simulink model "Model"  (R2020b)
settings: Solver=FixedStepDiscrete  StartTime=0.0  StopTime=inf  RelTol=1e-3
undefined symbols (not defined in the file): C12, designMultirateFIR, dt0
libraries: dspmlti4 x96, dspsrcs4 x89
(part 3 of 6)

== system Model/CORE_3_5/Path5 ==
  <IQ> : Inport
  Complex to Real-Imag : ComplexToRealImag
  Complex to Real-Imag1 : ComplexToRealImag
  Constant : Constant  Value=C12  SampleTime=dt0
  DDS_Gen1 : Subsystem
  FIR Dec1 : dspmlti4/FIR Decimation  FilterSource=Input port  h=designMultirateFIR(1,2)  D=2  filtStruct=Direct form  FilterObject=FDECIM  framing=Allow multirate processing  inputOffset=0  outputBufInitCond=0  roundingMode=Floor  overflowMode=off  firstCoeffDataTypeStr=Inherit: Same word length as input  firstCoeffMin=[]  firstCoeffMax=[]  firstCoeffLastDataTypeStr=Inherit: Same word length as input  outputDataTypeStr=Inherit: Same as accumulator  outputMin=[]  outputMax=[]  outputLastDataTypeStr=Inherit: Same as accumulator
  Freq1 : Constant  Value=2.4e6
  Mixer1 : Subsystem
  Real-Imag to Complex : RealImagToComplex
  Out1 : Outport
  wires:
  Constant/1 -> FIR Dec1/2
  Complex to Real-Imag/1 -> Mixer1/1(Input_I)
  Complex to Real-Imag1/1 -> Mixer1/3(DDS_I)
  Mixer1/2(Output_Q) -> Real-Imag to Complex/2
  Freq1/1 -> DDS_Gen1/1(In1)
  Complex to Real-Imag/2 -> Mixer1/2(Input_Q)
  Complex to Real-Imag1/2 -> Mixer1/4(DDS_Q)
  DDS_Gen1/1(Out1) -> Complex to Real-Imag1/1
  Real-Imag to Complex/1 -> FIR Dec1/1
  Mixer1/1(Output_I) -> Real-Imag to Complex/1
  FIR Dec1/1 -> Out1/1
  <IQ>/1 -> Complex to Real-Imag/1

== system Model/CORE_3_5/Path6 ==
  <IQ> : Inport
  Complex to Real-Imag : ComplexToRealImag
  Complex to Real-Imag1 : ComplexToRealImag
  Constant : Constant  Value=C12  SampleTime=dt0
  DDS_Gen1 : Subsystem
  FIR Dec1 : dspmlti4/FIR Decimation  FilterSource=Input port  h=designMultirateFIR(1,2)  D=2  filtStruct=Direct form  FilterObject=FDECIM  framing=Allow multirate processing  inputOffset=0  outputBufInitCond=0  roundingMode=Floor  overflowMode=off  firstCoeffDataTypeStr=Inherit: Same word length as input  firstCoeffMin=[]  firstCoeffMax=[]  firstCoeffLastDataTypeStr=Inherit: Same word length as input  outputDataTypeStr=Inherit: Same as accumulator  outputMin=[]  outputMax=[]  outputLastDataTypeStr=Inherit: Same as accumulator
  Freq1 : Constant  Value=2.4e6
  Mixer1 : Subsystem
  Real-Imag to Complex : RealImagToComplex
  Out1 : Outport
  wires:
  Constant/1 -> FIR Dec1/2
  Complex to Real-Imag/1 -> Mixer1/1(Input_I)
  Complex to Real-Imag1/1 -> Mixer1/3(DDS_I)
  Mixer1/2(Output_Q) -> Real-Imag to Complex/2
  Freq1/1 -> DDS_Gen1/1(In1)
  Complex to Real-Imag/2 -> Mixer1/2(Input_Q)
  Complex to Real-Imag1/2 -> Mixer1/4(DDS_Q)
  DDS_Gen1/1(Out1) -> Complex to Real-Imag1/1
  Real-Imag to Complex/1 -> FIR Dec1/1
  Mixer1/1(Output_I) -> Real-Imag to Complex/1
  FIR Dec1/1 -> Out1/1
  <IQ>/1 -> Complex to Real-Imag/1

== system Model/CORE_3_5/Path7 ==
  <IQ> : Inport
  Complex to Real-Imag : ComplexToRealImag
  Complex to Real-Imag1 : ComplexToRealImag
  Constant : Constant  Value=C12  SampleTime=dt0
  DDS_Gen1 : Subsystem
  FIR Dec1 : dspmlti4/FIR Decimation  FilterSource=Input port  h=designMultirateFIR(1,2)  D=2  filtStruct=Direct form  FilterObject=FDECIM  framing=Allow multirate processing  inputOffset=0  outputBufInitCond=0  roundingMode=Floor  overflowMode=off  firstCoeffDataTypeStr=Inherit: Same word length as input  firstCoeffMin=[]  firstCoeffMax=[]  firstCoeffLastDataTypeStr=Inherit: Same word length as input  outputDataTypeStr=Inherit: Same as accumulator  outputMin=[]  outputMax=[]  outputLastDataTypeStr=Inherit: Same as accumulator
  Freq1 : Constant  Value=2.4e6
  Mixer1 : Subsystem
  Real-Imag to Complex : RealImagToComplex
  Out1 : Outport
  wires:
  Constant/1 -> FIR Dec1/2
  Complex to Real-Imag/1 -> Mixer1/1(Input_I)
  Complex to Real-Imag1/1 -> Mixer1/3(DDS_I)
  Mixer1/2(Output_Q) -> Real-Imag to Complex/2
  Freq1/1 -> DDS_Gen1/1(In1)
  Complex to Real-Imag/2 -> Mixer1/2(Input_Q)
  Complex to Real-Imag1/2 -> Mixer1/4(DDS_Q)
  DDS_Gen1/1(Out1) -> Complex to Real-Imag1/1
  Real-Imag to Complex/1 -> FIR Dec1/1
  Mixer1/1(Output_I) -> Real-Imag to Complex/1
  FIR Dec1/1 -> Out1/1
  <IQ>/1 -> Complex to Real-Imag/1

== system Model/CORE_3_5/Path8 ==
  <IQ> : Inport
  Complex to Real-Imag : ComplexToRealImag
  Complex to Real-Imag1 : ComplexToRealImag
  Constant : Constant  Value=C12  SampleTime=dt0
  DDS_Gen1 : Subsystem
  FIR Dec1 : dspmlti4/FIR Decimation  FilterSource=Input port  h=designMultirateFIR(1,2)  D=2  filtStruct=Direct form  FilterObject=FDECIM  framing=Allow multirate processing  inputOffset=0  outputBufInitCond=0  roundingMode=Floor  overflowMode=off  firstCoeffDataTypeStr=Inherit: Same word length as input  firstCoeffMin=[]  firstCoeffMax=[]  firstCoeffLastDataTypeStr=Inherit: Same word length as input  outputDataTypeStr=Inherit: Same as accumulator  outputMin=[]  outputMax=[]  outputLastDataTypeStr=Inherit: Same as accumulator
  Freq1 : Constant  Value=2.4e6
  Mixer1 : Subsystem
  Real-Imag to Complex : RealImagToComplex
  Out1 : Outport
  wires:
  Constant/1 -> FIR Dec1/2
  Complex to Real-Imag/1 -> Mixer1/1(Input_I)
  Complex to Real-Imag1/1 -> Mixer1/3(DDS_I)
  Mixer1/2(Output_Q) -> Real-Imag to Complex/2
  Freq1/1 -> DDS_Gen1/1(In1)
  Complex to Real-Imag/2 -> Mixer1/2(Input_Q)
  Complex to Real-Imag1/2 -> Mixer1/4(DDS_Q)
  DDS_Gen1/1(Out1) -> Complex to Real-Imag1/1
  Real-Imag to Complex/1 -> FIR Dec1/1
  Mixer1/1(Output_I) -> Real-Imag to Complex/1
  FIR Dec1/1 -> Out1/1
  <IQ>/1 -> Complex to Real-Imag/1

== system Model/CORE_3_6/Path1 ==
  <IQ> : Inport
  Complex to Real-Imag : ComplexToRealImag
  Complex to Real-Imag1 : ComplexToRealImag
  Constant : Constant  Value=C12  SampleTime=dt0
  DDS_Gen1 : Subsystem
  FIR Dec1 : dspmlti4/FIR Decimation  FilterSource=Input port  h=designMultirateFIR(1,2)  D=2  filtStruct=Direct form  FilterObject=FDECIM  framing=Allow multirate processing  inputOffset=0  outputBufInitCond=0  roundingMode=Floor  overflowMode=off  firstCoeffDataTypeStr=Inherit: Same word length as input  firstCoeffMin=[]  firstCoeffMax=[]  firstCoeffLastDataTypeStr=Inherit: Same word length as input  outputDataTypeStr=Inherit: Same as accumulator  outputMin=[]  outputMax=[]  outputLastDataTypeStr=Inherit: Same as accumulator
  Freq1 : Constant  Value=2.4e6
  Mixer1 : Subsystem
  Real-Imag to Complex : RealImagToComplex
  Out1 : Outport
  wires:
  Constant/1 -> FIR Dec1/2
  Complex to Real-Imag/1 -> Mixer1/1(Input_I)
  Complex to Real-Imag1/1 -> Mixer1/3(DDS_I)
  Mixer1/2(Output_Q) -> Real-Imag to Complex/2
  Freq1/1 -> DDS_Gen1/1(In1)
  Complex to Real-Imag/2 -> Mixer1/2(Input_Q)
  Complex to Real-Imag1/2 -> Mixer1/4(DDS_Q)
  DDS_Gen1/1(Out1) -> Complex to Real-Imag1/1
  Real-Imag to Complex/1 -> FIR Dec1/1
  Mixer1/1(Output_I) -> Real-Imag to Complex/1
  FIR Dec1/1 -> Out1/1
  <IQ>/1 -> Complex to Real-Imag/1

== system Model/CORE_3_6/Path2 ==
  <IQ> : Inport
  Complex to Real-Imag : ComplexToRealImag
  Complex to Real-Imag1 : ComplexToRealImag
  Constant : Constant  Value=C12  SampleTime=dt0
  DDS_Gen1 : Subsystem
  FIR Dec1 : dspmlti4/FIR Decimation  FilterSource=Input port  h=designMultirateFIR(1,2)  D=2  filtStruct=Direct form  FilterObject=FDECIM  framing=Allow multirate processing  inputOffset=0  outputBufInitCond=0  roundingMode=Floor  overflowMode=off  firstCoeffDataTypeStr=Inherit: Same word length as input  firstCoeffMin=[]  firstCoeffMax=[]  firstCoeffLastDataTypeStr=Inherit: Same word length as input  outputDataTypeStr=Inherit: Same as accumulator  outputMin=[]  outputMax=[]  outputLastDataTypeStr=Inherit: Same as accumulator
  Freq1 : Constant  Value=2.4e6
  Mixer1 : Subsystem
  Real-Imag to Complex : RealImagToComplex
  Out1 : Outport
  wires:
  Constant/1 -> FIR Dec1/2
  Complex to Real-Imag/1 -> Mixer1/1(Input_I)
  Complex to Real-Imag1/1 -> Mixer1/3(DDS_I)
  Mixer1/2(Output_Q) -> Real-Imag to Complex/2
  Freq1/1 -> DDS_Gen1/1(In1)
  Complex to Real-Imag/2 -> Mixer1/2(Input_Q)
  Complex to Real-Imag1/2 -> Mixer1/4(DDS_Q)
  DDS_Gen1/1(Out1) -> Complex to Real-Imag1/1
  Real-Imag to Complex/1 -> FIR Dec1/1
  Mixer1/1(Output_I) -> Real-Imag to Complex/1
  FIR Dec1/1 -> Out1/1
  <IQ>/1 -> Complex to Real-Imag/1

== system Model/CORE_3_6/Path3 ==
  <IQ> : Inport
  Complex to Real-Imag : ComplexToRealImag
  Complex to Real-Imag1 : ComplexToRealImag
  Constant : Constant  Value=C12  SampleTime=dt0
  DDS_Gen1 : Subsystem
  FIR Dec1 : dspmlti4/FIR Decimation  FilterSource=Input port  h=designMultirateFIR(1,2)  D=2  filtStruct=Direct form  FilterObject=FDECIM  framing=Allow multirate processing  inputOffset=0  outputBufInitCond=0  roundingMode=Floor  overflowMode=off  firstCoeffDataTypeStr=Inherit: Same word length as input  firstCoeffMin=[]  firstCoeffMax=[]  firstCoeffLastDataTypeStr=Inherit: Same word length as input  outputDataTypeStr=Inherit: Same as accumulator  outputMin=[]  outputMax=[]  outputLastDataTypeStr=Inherit: Same as accumulator
  Freq1 : Constant  Value=2.4e6
  Mixer1 : Subsystem
  Real-Imag to Complex : RealImagToComplex
  Out1 : Outport
  wires:
  Constant/1 -> FIR Dec1/2
  Complex to Real-Imag/1 -> Mixer1/1(Input_I)
  Complex to Real-Imag1/1 -> Mixer1/3(DDS_I)
  Mixer1/2(Output_Q) -> Real-Imag to Complex/2
  Freq1/1 -> DDS_Gen1/1(In1)
  Complex to Real-Imag/2 -> Mixer1/2(Input_Q)
  Complex to Real-Imag1/2 -> Mixer1/4(DDS_Q)
  DDS_Gen1/1(Out1) -> Complex to Real-Imag1/1
  Real-Imag to Complex/1 -> FIR Dec1/1
  Mixer1/1(Output_I) -> Real-Imag to Complex/1
  FIR Dec1/1 -> Out1/1
  <IQ>/1 -> Complex to Real-Imag/1

== system Model/CORE_3_6/Path4 ==
  <IQ> : Inport
  Complex to Real-Imag : ComplexToRealImag
  Complex to Real-Imag1 : ComplexToRealImag
  Constant : Constant  Value=C12  SampleTime=dt0
  DDS_Gen1 : Subsystem
  FIR Dec1 : dspmlti4/FIR Decimation  FilterSource=Input port  h=designMultirateFIR(1,2)  D=2  filtStruct=Direct form  FilterObject=FDECIM  framing=Allow multirate processing  inputOffset=0  outputBufInitCond=0  roundingMode=Floor  overflowMode=off  firstCoeffDataTypeStr=Inherit: Same word length as input  firstCoeffMin=[]  firstCoeffMax=[]  firstCoeffLastDataTypeStr=Inherit: Same word length as input  outputDataTypeStr=Inherit: Same as accumulator  outputMin=[]  outputMax=[]  outputLastDataTypeStr=Inherit: Same as accumulator
  Freq1 : Constant  Value=2.4e6
  Mixer1 : Subsystem
  Real-Imag to Complex : RealImagToComplex
  Out1 : Outport
  wires:
  Constant/1 -> FIR Dec1/2
  Complex to Real-Imag/1 -> Mixer1/1(Input_I)
  Complex to Real-Imag1/1 -> Mixer1/3(DDS_I)
  Mixer1/2(Output_Q) -> Real-Imag to Complex/2
  Freq1/1 -> DDS_Gen1/1(In1)
  Complex to Real-Imag/2 -> Mixer1/2(Input_Q)
  Complex to Real-Imag1/2 -> Mixer1/4(DDS_Q)
  DDS_Gen1/1(Out1) -> Complex to Real-Imag1/1
  Real-Imag to Complex/1 -> FIR Dec1/1
  Mixer1/1(Output_I) -> Real-Imag to Complex/1
  FIR Dec1/1 -> Out1/1
  <IQ>/1 -> Complex to Real-Imag/1

== system Model/CORE_3_6/Path5 ==
  <IQ> : Inport
  Complex to Real-Imag : ComplexToRealImag
  Complex to Real-Imag1 : ComplexToRealImag
  Constant : Constant  Value=C12  SampleTime=dt0
  DDS_Gen1 : Subsystem
  FIR Dec1 : dspmlti4/FIR Decimation  FilterSource=Input port  h=designMultirateFIR(1,2)  D=2  filtStruct=Direct form  FilterObject=FDECIM  framing=Allow multirate processing  inputOffset=0  outputBufInitCond=0  roundingMode=Floor  overflowMode=off  firstCoeffDataTypeStr=Inherit: Same word length as input  firstCoeffMin=[]  firstCoeffMax=[]  firstCoeffLastDataTypeStr=Inherit: Same word length as input  outputDataTypeStr=Inherit: Same as accumulator  outputMin=[]  outputMax=[]  outputLastDataTypeStr=Inherit: Same as accumulator
  Freq1 : Constant  Value=2.4e6
  Mixer1 : Subsystem
  Real-Imag to Complex : RealImagToComplex
  Out1 : Outport
  wires:
  Constant/1 -> FIR Dec1/2
  Complex to Real-Imag/1 -> Mixer1/1(Input_I)
  Complex to Real-Imag1/1 -> Mixer1/3(DDS_I)
  Mixer1/2(Output_Q) -> Real-Imag to Complex/2
  Freq1/1 -> DDS_Gen1/1(In1)
  Complex to Real-Imag/2 -> Mixer1/2(Input_Q)
  Complex to Real-Imag1/2 -> Mixer1/4(DDS_Q)
  DDS_Gen1/1(Out1) -> Complex to Real-Imag1/1
  Real-Imag to Complex/1 -> FIR Dec1/1
  Mixer1/1(Output_I) -> Real-Imag to Complex/1
  FIR Dec1/1 -> Out1/1
  <IQ>/1 -> Complex to Real-Imag/1

== system Model/CORE_3_6/Path6 ==
  <IQ> : Inport
  Complex to Real-Imag : ComplexToRealImag
  Complex to Real-Imag1 : ComplexToRealImag
  Constant : Constant  Value=C12  SampleTime=dt0
  DDS_Gen1 : Subsystem
  FIR Dec1 : dspmlti4/FIR Decimation  FilterSource=Input port  h=designMultirateFIR(1,2)  D=2  filtStruct=Direct form  FilterObject=FDECIM  framing=Allow multirate processing  inputOffset=0  outputBufInitCond=0  roundingMode=Floor  overflowMode=off  firstCoeffDataTypeStr=Inherit: Same word length as input  firstCoeffMin=[]  firstCoeffMax=[]  firstCoeffLastDataTypeStr=Inherit: Same word length as input  outputDataTypeStr=Inherit: Same as accumulator  outputMin=[]  outputMax=[]  outputLastDataTypeStr=Inherit: Same as accumulator
  Freq1 : Constant  Value=2.4e6
  Mixer1 : Subsystem
  Real-Imag to Complex : RealImagToComplex
  Out1 : Outport
  wires:
  Constant/1 -> FIR Dec1/2
  Complex to Real-Imag/1 -> Mixer1/1(Input_I)
  Complex to Real-Imag1/1 -> Mixer1/3(DDS_I)
  Mixer1/2(Output_Q) -> Real-Imag to Complex/2
  Freq1/1 -> DDS_Gen1/1(In1)
  Complex to Real-Imag/2 -> Mixer1/2(Input_Q)
  Complex to Real-Imag1/2 -> Mixer1/4(DDS_Q)
  DDS_Gen1/1(Out1) -> Complex to Real-Imag1/1
  Real-Imag to Complex/1 -> FIR Dec1/1
  Mixer1/1(Output_I) -> Real-Imag to Complex/1
  FIR Dec1/1 -> Out1/1
  <IQ>/1 -> Complex to Real-Imag/1

== system Model/CORE_3_6/Path7 ==
  <IQ> : Inport
  Complex to Real-Imag : ComplexToRealImag
  Complex to Real-Imag1 : ComplexToRealImag
  Constant : Constant  Value=C12  SampleTime=dt0
  DDS_Gen1 : Subsystem
  FIR Dec1 : dspmlti4/FIR Decimation  FilterSource=Input port  h=designMultirateFIR(1,2)  D=2  filtStruct=Direct form  FilterObject=FDECIM  framing=Allow multirate processing  inputOffset=0  outputBufInitCond=0  roundingMode=Floor  overflowMode=off  firstCoeffDataTypeStr=Inherit: Same word length as input  firstCoeffMin=[]  firstCoeffMax=[]  firstCoeffLastDataTypeStr=Inherit: Same word length as input  outputDataTypeStr=Inherit: Same as accumulator  outputMin=[]  outputMax=[]  outputLastDataTypeStr=Inherit: Same as accumulator
  Freq1 : Constant  Value=2.4e6
  Mixer1 : Subsystem
  Real-Imag to Complex : RealImagToComplex
  Out1 : Outport
  wires:
  Constant/1 -> FIR Dec1/2
  Complex to Real-Imag/1 -> Mixer1/1(Input_I)
  Complex to Real-Imag1/1 -> Mixer1/3(DDS_I)
  Mixer1/2(Output_Q) -> Real-Imag to Complex/2
  Freq1/1 -> DDS_Gen1/1(In1)
  Complex to Real-Imag/2 -> Mixer1/2(Input_Q)
  Complex to Real-Imag1/2 -> Mixer1/4(DDS_Q)
  DDS_Gen1/1(Out1) -> Complex to Real-Imag1/1
  Real-Imag to Complex/1 -> FIR Dec1/1
  Mixer1/1(Output_I) -> Real-Imag to Complex/1
  FIR Dec1/1 -> Out1/1
  <IQ>/1 -> Complex to Real-Imag/1

== system Model/CORE_3_6/Path8 ==
  <IQ> : Inport
  Complex to Real-Imag : ComplexToRealImag
  Complex to Real-Imag1 : ComplexToRealImag
  Constant : Constant  Value=C12  SampleTime=dt0
  DDS_Gen1 : Subsystem
  FIR Dec1 : dspmlti4/FIR Decimation  FilterSource=Input port  h=designMultirateFIR(1,2)  D=2  filtStruct=Direct form  FilterObject=FDECIM  framing=Allow multirate processing  inputOffset=0  outputBufInitCond=0  roundingMode=Floor  overflowMode=off  firstCoeffDataTypeStr=Inherit: Same word length as input  firstCoeffMin=[]  firstCoeffMax=[]  firstCoeffLastDataTypeStr=Inherit: Same word length as input  outputDataTypeStr=Inherit: Same as accumulator  outputMin=[]  outputMax=[]  outputLastDataTypeStr=Inherit: Same as accumulator
  Freq1 : Constant  Value=2.4e6
  Mixer1 : Subsystem
  Real-Imag to Complex : RealImagToComplex
  Out1 : Outport
  wires:
  Constant/1 -> FIR Dec1/2
  Complex to Real-Imag/1 -> Mixer1/1(Input_I)
  Complex to Real-Imag1/1 -> Mixer1/3(DDS_I)
  Mixer1/2(Output_Q) -> Real-Imag to Complex/2
  Freq1/1 -> DDS_Gen1/1(In1)
  Complex to Real-Imag/2 -> Mixer1/2(Input_Q)
  Complex to Real-Imag1/2 -> Mixer1/4(DDS_Q)
  DDS_Gen1/1(Out1) -> Complex to Real-Imag1/1
  Real-Imag to Complex/1 -> FIR Dec1/1
  Mixer1/1(Output_I) -> Real-Imag to Complex/1
  FIR Dec1/1 -> Out1/1
  <IQ>/1 -> Complex to Real-Imag/1

== system Model/CORE_3_7/Path1 ==
  <IQ> : Inport
  Complex to Real-Imag : ComplexToRealImag
  Complex to Real-Imag1 : ComplexToRealImag
  Constant : Constant  Value=C12  SampleTime=dt0
  DDS_Gen1 : Subsystem
  FIR Dec1 : dspmlti4/FIR Decimation  FilterSource=Input port  h=designMultirateFIR(1,2)  D=2  filtStruct=Direct form  FilterObject=FDECIM  framing=Allow multirate processing  inputOffset=0  outputBufInitCond=0  roundingMode=Floor  overflowMode=off  firstCoeffDataTypeStr=Inherit: Same word length as input  firstCoeffMin=[]  firstCoeffMax=[]  firstCoeffLastDataTypeStr=Inherit: Same word length as input  outputDataTypeStr=Inherit: Same as accumulator  outputMin=[]  outputMax=[]  outputLastDataTypeStr=Inherit: Same as accumulator
  Freq1 : Constant  Value=2.4e6
  Mixer1 : Subsystem
  Real-Imag to Complex : RealImagToComplex
  Out1 : Outport
  wires:
  Constant/1 -> FIR Dec1/2
  Complex to Real-Imag/1 -> Mixer1/1(Input_I)
  Complex to Real-Imag1/1 -> Mixer1/3(DDS_I)
  Mixer1/2(Output_Q) -> Real-Imag to Complex/2
  Freq1/1 -> DDS_Gen1/1(In1)
  Complex to Real-Imag/2 -> Mixer1/2(Input_Q)
  Complex to Real-Imag1/2 -> Mixer1/4(DDS_Q)
  DDS_Gen1/1(Out1) -> Complex to Real-Imag1/1
  Real-Imag to Complex/1 -> FIR Dec1/1
  Mixer1/1(Output_I) -> Real-Imag to Complex/1
  FIR Dec1/1 -> Out1/1
  <IQ>/1 -> Complex to Real-Imag/1

== system Model/CORE_3_7/Path2 ==
  <IQ> : Inport
  Complex to Real-Imag : ComplexToRealImag
  Complex to Real-Imag1 : ComplexToRealImag
  Constant : Constant  Value=C12  SampleTime=dt0
  DDS_Gen1 : Subsystem
  FIR Dec1 : dspmlti4/FIR Decimation  FilterSource=Input port  h=designMultirateFIR(1,2)  D=2  filtStruct=Direct form  FilterObject=FDECIM  framing=Allow multirate processing  inputOffset=0  outputBufInitCond=0  roundingMode=Floor  overflowMode=off  firstCoeffDataTypeStr=Inherit: Same word length as input  firstCoeffMin=[]  firstCoeffMax=[]  firstCoeffLastDataTypeStr=Inherit: Same word length as input  outputDataTypeStr=Inherit: Same as accumulator  outputMin=[]  outputMax=[]  outputLastDataTypeStr=Inherit: Same as accumulator
  Freq1 : Constant  Value=2.4e6
  Mixer1 : Subsystem
  Real-Imag to Complex : RealImagToComplex
  Out1 : Outport
  wires:
  Constant/1 -> FIR Dec1/2
  Complex to Real-Imag/1 -> Mixer1/1(Input_I)
  Complex to Real-Imag1/1 -> Mixer1/3(DDS_I)
  Mixer1/2(Output_Q) -> Real-Imag to Complex/2
  Freq1/1 -> DDS_Gen1/1(In1)
  Complex to Real-Imag/2 -> Mixer1/2(Input_Q)
  Complex to Real-Imag1/2 -> Mixer1/4(DDS_Q)
  DDS_Gen1/1(Out1) -> Complex to Real-Imag1/1
  Real-Imag to Complex/1 -> FIR Dec1/1
  Mixer1/1(Output_I) -> Real-Imag to Complex/1
  FIR Dec1/1 -> Out1/1
  <IQ>/1 -> Complex to Real-Imag/1

== system Model/CORE_3_7/Path3 ==
  <IQ> : Inport
  Complex to Real-Imag : ComplexToRealImag
  Complex to Real-Imag1 : ComplexToRealImag
  Constant : Constant  Value=C12  SampleTime=dt0
  DDS_Gen1 : Subsystem
  FIR Dec1 : dspmlti4/FIR Decimation  FilterSource=Input port  h=designMultirateFIR(1,2)  D=2  filtStruct=Direct form  FilterObject=FDECIM  framing=Allow multirate processing  inputOffset=0  outputBufInitCond=0  roundingMode=Floor  overflowMode=off  firstCoeffDataTypeStr=Inherit: Same word length as input  firstCoeffMin=[]  firstCoeffMax=[]  firstCoeffLastDataTypeStr=Inherit: Same word length as input  outputDataTypeStr=Inherit: Same as accumulator  outputMin=[]  outputMax=[]  outputLastDataTypeStr=Inherit: Same as accumulator
  Freq1 : Constant  Value=2.4e6
  Mixer1 : Subsystem
  Real-Imag to Complex : RealImagToComplex
  Out1 : Outport
  wires:
  Constant/1 -> FIR Dec1/2
  Complex to Real-Imag/1 -> Mixer1/1(Input_I)
  Complex to Real-Imag1/1 -> Mixer1/3(DDS_I)
  Mixer1/2(Output_Q) -> Real-Imag to Complex/2
  Freq1/1 -> DDS_Gen1/1(In1)
  Complex to Real-Imag/2 -> Mixer1/2(Input_Q)
  Complex to Real-Imag1/2 -> Mixer1/4(DDS_Q)
  DDS_Gen1/1(Out1) -> Complex to Real-Imag1/1
  Real-Imag to Complex/1 -> FIR Dec1/1
  Mixer1/1(Output_I) -> Real-Imag to Complex/1
  FIR Dec1/1 -> Out1/1
  <IQ>/1 -> Complex to Real-Imag/1

== system Model/CORE_3_7/Path4 ==
  <IQ> : Inport
  Complex to Real-Imag : ComplexToRealImag
  Complex to Real-Imag1 : ComplexToRealImag
  Constant : Constant  Value=C12  SampleTime=dt0
  DDS_Gen1 : Subsystem
  FIR Dec1 : dspmlti4/FIR Decimation  FilterSource=Input port  h=designMultirateFIR(1,2)  D=2  filtStruct=Direct form  FilterObject=FDECIM  framing=Allow multirate processing  inputOffset=0  outputBufInitCond=0  roundingMode=Floor  overflowMode=off  firstCoeffDataTypeStr=Inherit: Same word length as input  firstCoeffMin=[]  firstCoeffMax=[]  firstCoeffLastDataTypeStr=Inherit: Same word length as input  outputDataTypeStr=Inherit: Same as accumulator  outputMin=[]  outputMax=[]  outputLastDataTypeStr=Inherit: Same as accumulator
  Freq1 : Constant  Value=2.4e6
  Mixer1 : Subsystem
  Real-Imag to Complex : RealImagToComplex
  Out1 : Outport
  wires:
  Constant/1 -> FIR Dec1/2
  Complex to Real-Imag/1 -> Mixer1/1(Input_I)
  Complex to Real-Imag1/1 -> Mixer1/3(DDS_I)
  Mixer1/2(Output_Q) -> Real-Imag to Complex/2
  Freq1/1 -> DDS_Gen1/1(In1)
  Complex to Real-Imag/2 -> Mixer1/2(Input_Q)
  Complex to Real-Imag1/2 -> Mixer1/4(DDS_Q)
  DDS_Gen1/1(Out1) -> Complex to Real-Imag1/1
  Real-Imag to Complex/1 -> FIR Dec1/1
  Mixer1/1(Output_I) -> Real-Imag to Complex/1
  FIR Dec1/1 -> Out1/1
  <IQ>/1 -> Complex to Real-Imag/1

== system Model/CORE_3_7/Path5 ==
  <IQ> : Inport
  Complex to Real-Imag : ComplexToRealImag
  Complex to Real-Imag1 : ComplexToRealImag
  Constant : Constant  Value=C12  SampleTime=dt0
  DDS_Gen1 : Subsystem
  FIR Dec1 : dspmlti4/FIR Decimation  FilterSource=Input port  h=designMultirateFIR(1,2)  D=2  filtStruct=Direct form  FilterObject=FDECIM  framing=Allow multirate processing  inputOffset=0  outputBufInitCond=0  roundingMode=Floor  overflowMode=off  firstCoeffDataTypeStr=Inherit: Same word length as input  firstCoeffMin=[]  firstCoeffMax=[]  firstCoeffLastDataTypeStr=Inherit: Same word length as input  outputDataTypeStr=Inherit: Same as accumulator  outputMin=[]  outputMax=[]  outputLastDataTypeStr=Inherit: Same as accumulator
  Freq1 : Constant  Value=2.4e6
  Mixer1 : Subsystem
  Real-Imag to Complex : RealImagToComplex
  Out1 : Outport
  wires:
  Constant/1 -> FIR Dec1/2
  Complex to Real-Imag/1 -> Mixer1/1(Input_I)
  Complex to Real-Imag1/1 -> Mixer1/3(DDS_I)
  Mixer1/2(Output_Q) -> Real-Imag to Complex/2
  Freq1/1 -> DDS_Gen1/1(In1)
  Complex to Real-Imag/2 -> Mixer1/2(Input_Q)
  Complex to Real-Imag1/2 -> Mixer1/4(DDS_Q)
  DDS_Gen1/1(Out1) -> Complex to Real-Imag1/1
  Real-Imag to Complex/1 -> FIR Dec1/1
  Mixer1/1(Output_I) -> Real-Imag to Complex/1
  FIR Dec1/1 -> Out1/1
  <IQ>/1 -> Complex to Real-Imag/1

== system Model/CORE_3_7/Path6 ==
  <IQ> : Inport
  Complex to Real-Imag : ComplexToRealImag
  Complex to Real-Imag1 : ComplexToRealImag
  Constant : Constant  Value=C12  SampleTime=dt0
  DDS_Gen1 : Subsystem
  FIR Dec1 : dspmlti4/FIR Decimation  FilterSource=Input port  h=designMultirateFIR(1,2)  D=2  filtStruct=Direct form  FilterObject=FDECIM  framing=Allow multirate processing  inputOffset=0  outputBufInitCond=0  roundingMode=Floor  overflowMode=off  firstCoeffDataTypeStr=Inherit: Same word length as input  firstCoeffMin=[]  firstCoeffMax=[]  firstCoeffLastDataTypeStr=Inherit: Same word length as input  outputDataTypeStr=Inherit: Same as accumulator  outputMin=[]  outputMax=[]  outputLastDataTypeStr=Inherit: Same as accumulator
  Freq1 : Constant  Value=2.4e6
  Mixer1 : Subsystem
  Real-Imag to Complex : RealImagToComplex
  Out1 : Outport
  wires:
  Constant/1 -> FIR Dec1/2
  Complex to Real-Imag/1 -> Mixer1/1(Input_I)
  Complex to Real-Imag1/1 -> Mixer1/3(DDS_I)
  Mixer1/2(Output_Q) -> Real-Imag to Complex/2
  Freq1/1 -> DDS_Gen1/1(In1)
  Complex to Real-Imag/2 -> Mixer1/2(Input_Q)
  Complex to Real-Imag1/2 -> Mixer1/4(DDS_Q)
  DDS_Gen1/1(Out1) -> Complex to Real-Imag1/1
  Real-Imag to Complex/1 -> FIR Dec1/1
  Mixer1/1(Output_I) -> Real-Imag to Complex/1
  FIR Dec1/1 -> Out1/1
  <IQ>/1 -> Complex to Real-Imag/1

== system Model/CORE_3_7/Path7 ==
  <IQ> : Inport
  Complex to Real-Imag : ComplexToRealImag
  Complex to Real-Imag1 : ComplexToRealImag
  Constant : Constant  Value=C12  SampleTime=dt0
  DDS_Gen1 : Subsystem
  FIR Dec1 : dspmlti4/FIR Decimation  FilterSource=Input port  h=designMultirateFIR(1,2)  D=2  filtStruct=Direct form  FilterObject=FDECIM  framing=Allow multirate processing  inputOffset=0  outputBufInitCond=0  roundingMode=Floor  overflowMode=off  firstCoeffDataTypeStr=Inherit: Same word length as input  firstCoeffMin=[]  firstCoeffMax=[]  firstCoeffLastDataTypeStr=Inherit: Same word length as input  outputDataTypeStr=Inherit: Same as accumulator  outputMin=[]  outputMax=[]  outputLastDataTypeStr=Inherit: Same as accumulator
  Freq1 : Constant  Value=2.4e6
  Mixer1 : Subsystem
  Real-Imag to Complex : RealImagToComplex
  Out1 : Outport
  wires:
  Constant/1 -> FIR Dec1/2
  Complex to Real-Imag/1 -> Mixer1/1(Input_I)
  Complex to Real-Imag1/1 -> Mixer1/3(DDS_I)
  Mixer1/2(Output_Q) -> Real-Imag to Complex/2
  Freq1/1 -> DDS_Gen1/1(In1)
  Complex to Real-Imag/2 -> Mixer1/2(Input_Q)
  Complex to Real-Imag1/2 -> Mixer1/4(DDS_Q)
  DDS_Gen1/1(Out1) -> Complex to Real-Imag1/1
  Real-Imag to Complex/1 -> FIR Dec1/1
  Mixer1/1(Output_I) -> Real-Imag to Complex/1
  FIR Dec1/1 -> Out1/1
  <IQ>/1 -> Complex to Real-Imag/1

== system Model/CORE_3_7/Path8 ==
  <IQ> : Inport
  Complex to Real-Imag : ComplexToRealImag
  Complex to Real-Imag1 : ComplexToRealImag
  Constant : Constant  Value=C12  SampleTime=dt0
  DDS_Gen1 : Subsystem
  FIR Dec1 : dspmlti4/FIR Decimation  FilterSource=Input port  h=designMultirateFIR(1,2)  D=2  filtStruct=Direct form  FilterObject=FDECIM  framing=Allow multirate processing  inputOffset=0  outputBufInitCond=0  roundingMode=Floor  overflowMode=off  firstCoeffDataTypeStr=Inherit: Same word length as input  firstCoeffMin=[]  firstCoeffMax=[]  firstCoeffLastDataTypeStr=Inherit: Same word length as input  outputDataTypeStr=Inherit: Same as accumulator  outputMin=[]  outputMax=[]  outputLastDataTypeStr=Inherit: Same as accumulator
  Freq1 : Constant  Value=2.4e6
  Mixer1 : Subsystem
  Real-Imag to Complex : RealImagToComplex
  Out1 : Outport
  wires:
  Constant/1 -> FIR Dec1/2
  Complex to Real-Imag/1 -> Mixer1/1(Input_I)
  Complex to Real-Imag1/1 -> Mixer1/3(DDS_I)
  Mixer1/2(Output_Q) -> Real-Imag to Complex/2
  Freq1/1 -> DDS_Gen1/1(In1)
  Complex to Real-Imag/2 -> Mixer1/2(Input_Q)
  Complex to Real-Imag1/2 -> Mixer1/4(DDS_Q)
  DDS_Gen1/1(Out1) -> Complex to Real-Imag1/1
  Real-Imag to Complex/1 -> FIR Dec1/1
  Mixer1/1(Output_I) -> Real-Imag to Complex/1
  FIR Dec1/1 -> Out1/1
  <IQ>/1 -> Complex to Real-Imag/1

== system Model/CORE_3_8/Path1 ==
  <IQ> : Inport
  Complex to Real-Imag : ComplexToRealImag
  Complex to Real-Imag1 : ComplexToRealImag
  Constant : Constant  Value=C12  SampleTime=dt0
  DDS_Gen1 : Subsystem
  FIR Dec1 : dspmlti4/FIR Decimation  FilterSource=Input port  h=designMultirateFIR(1,2)  D=2  filtStruct=Direct form  FilterObject=FDECIM  framing=Allow multirate processing  inputOffset=0  outputBufInitCond=0  roundingMode=Floor  overflowMode=off  firstCoeffDataTypeStr=Inherit: Same word length as input  firstCoeffMin=[]  firstCoeffMax=[]  firstCoeffLastDataTypeStr=Inherit: Same word length as input  outputDataTypeStr=Inherit: Same as accumulator  outputMin=[]  outputMax=[]  outputLastDataTypeStr=Inherit: Same as accumulator
  Freq1 : Constant  Value=2.4e6
  Mixer1 : Subsystem
  Real-Imag to Complex : RealImagToComplex
  Out1 : Outport
  wires:
  Constant/1 -> FIR Dec1/2
  Complex to Real-Imag/1 -> Mixer1/1(Input_I)
  Complex to Real-Imag1/1 -> Mixer1/3(DDS_I)
  Mixer1/2(Output_Q) -> Real-Imag to Complex/2
  Freq1/1 -> DDS_Gen1/1(In1)
  Complex to Real-Imag/2 -> Mixer1/2(Input_Q)
  Complex to Real-Imag1/2 -> Mixer1/4(DDS_Q)
  DDS_Gen1/1(Out1) -> Complex to Real-Imag1/1
  Real-Imag to Complex/1 -> FIR Dec1/1
  Mixer1/1(Output_I) -> Real-Imag to Complex/1
  FIR Dec1/1 -> Out1/1
  <IQ>/1 -> Complex to Real-Imag/1

== system Model/CORE_3_8/Path2 ==
  <IQ> : Inport
  Complex to Real-Imag : ComplexToRealImag
  Complex to Real-Imag1 : ComplexToRealImag
  Constant : Constant  Value=C12  SampleTime=dt0
  DDS_Gen1 : Subsystem
  FIR Dec1 : dspmlti4/FIR Decimation  FilterSource=Input port  h=designMultirateFIR(1,2)  D=2  filtStruct=Direct form  FilterObject=FDECIM  framing=Allow multirate processing  inputOffset=0  outputBufInitCond=0  roundingMode=Floor  overflowMode=off  firstCoeffDataTypeStr=Inherit: Same word length as input  firstCoeffMin=[]  firstCoeffMax=[]  firstCoeffLastDataTypeStr=Inherit: Same word length as input  outputDataTypeStr=Inherit: Same as accumulator  outputMin=[]  outputMax=[]  outputLastDataTypeStr=Inherit: Same as accumulator
  Freq1 : Constant  Value=2.4e6
  Mixer1 : Subsystem
  Real-Imag to Complex : RealImagToComplex
  Out1 : Outport
  wires:
  Constant/1 -> FIR Dec1/2
  Complex to Real-Imag/1 -> Mixer1/1(Input_I)
  Complex to Real-Imag1/1 -> Mixer1/3(DDS_I)
  Mixer1/2(Output_Q) -> Real-Imag to Complex/2
  Freq1/1 -> DDS_Gen1/1(In1)
  Complex to Real-Imag/2 -> Mixer1/2(Input_Q)
  Complex to Real-Imag1/2 -> Mixer1/4(DDS_Q)
  DDS_Gen1/1(Out1) -> Complex to Real-Imag1/1
  Real-Imag to Complex/1 -> FIR Dec1/1
  Mixer1/1(Output_I) -> Real-Imag to Complex/1
  FIR Dec1/1 -> Out1/1
  <IQ>/1 -> Complex to Real-Imag/1

== system Model/CORE_3_8/Path3 ==
  <IQ> : Inport
  Complex to Real-Imag : ComplexToRealImag
  Complex to Real-Imag1 : ComplexToRealImag
  Constant : Constant  Value=C12  SampleTime=dt0
  DDS_Gen1 : Subsystem
  FIR Dec1 : dspmlti4/FIR Decimation  FilterSource=Input port  h=designMultirateFIR(1,2)  D=2  filtStruct=Direct form  FilterObject=FDECIM  framing=Allow multirate processing  inputOffset=0  outputBufInitCond=0  roundingMode=Floor  overflowMode=off  firstCoeffDataTypeStr=Inherit: Same word length as input  firstCoeffMin=[]  firstCoeffMax=[]  firstCoeffLastDataTypeStr=Inherit: Same word length as input  outputDataTypeStr=Inherit: Same as accumulator  outputMin=[]  outputMax=[]  outputLastDataTypeStr=Inherit: Same as accumulator
  Freq1 : Constant  Value=2.4e6
  Mixer1 : Subsystem
  Real-Imag to Complex : RealImagToComplex
  Out1 : Outport
  wires:
  Constant/1 -> FIR Dec1/2
  Complex to Real-Imag/1 -> Mixer1/1(Input_I)
  Complex to Real-Imag1/1 -> Mixer1/3(DDS_I)
  Mixer1/2(Output_Q) -> Real-Imag to Complex/2
  Freq1/1 -> DDS_Gen1/1(In1)
  Complex to Real-Imag/2 -> Mixer1/2(Input_Q)
  Complex to Real-Imag1/2 -> Mixer1/4(DDS_Q)
  DDS_Gen1/1(Out1) -> Complex to Real-Imag1/1
  Real-Imag to Complex/1 -> FIR Dec1/1
  Mixer1/1(Output_I) -> Real-Imag to Complex/1
  FIR Dec1/1 -> Out1/1
  <IQ>/1 -> Complex to Real-Imag/1

== system Model/CORE_3_8/Path4 ==
  <IQ> : Inport
  Complex to Real-Imag : ComplexToRealImag
  Complex to Real-Imag1 : ComplexToRealImag
  Constant : Constant  Value=C12  SampleTime=dt0
  DDS_Gen1 : Subsystem
  FIR Dec1 : dspmlti4/FIR Decimation  FilterSource=Input port  h=designMultirateFIR(1,2)  D=2  filtStruct=Direct form  FilterObject=FDECIM  framing=Allow multirate processing  inputOffset=0  outputBufInitCond=0  roundingMode=Floor  overflowMode=off  firstCoeffDataTypeStr=Inherit: Same word length as input  firstCoeffMin=[]  firstCoeffMax=[]  firstCoeffLastDataTypeStr=Inherit: Same word length as input  outputDataTypeStr=Inherit: Same as accumulator  outputMin=[]  outputMax=[]  outputLastDataTypeStr=Inherit: Same as accumulator
  Freq1 : Constant  Value=2.4e6
  Mixer1 : Subsystem
  Real-Imag to Complex : RealImagToComplex
  Out1 : Outport
  wires:
  Constant/1 -> FIR Dec1/2
  Complex to Real-Imag/1 -> Mixer1/1(Input_I)
  Complex to Real-Imag1/1 -> Mixer1/3(DDS_I)
  Mixer1/2(Output_Q) -> Real-Imag to Complex/2
  Freq1/1 -> DDS_Gen1/1(In1)
  Complex to Real-Imag/2 -> Mixer1/2(Input_Q)
  Complex to Real-Imag1/2 -> Mixer1/4(DDS_Q)
  DDS_Gen1/1(Out1) -> Complex to Real-Imag1/1
  Real-Imag to Complex/1 -> FIR Dec1/1
  Mixer1/1(Output_I) -> Real-Imag to Complex/1
  FIR Dec1/1 -> Out1/1
  <IQ>/1 -> Complex to Real-Imag/1

== system Model/CORE_3_8/Path5 ==
  <IQ> : Inport
  Complex to Real-Imag : ComplexToRealImag
  Complex to Real-Imag1 : ComplexToRealImag
  Constant : Constant  Value=C12  SampleTime=dt0
  DDS_Gen1 : Subsystem
  FIR Dec1 : dspmlti4/FIR Decimation  FilterSource=Input port  h=designMultirateFIR(1,2)  D=2  filtStruct=Direct form  FilterObject=FDECIM  framing=Allow multirate processing  inputOffset=0  outputBufInitCond=0  roundingMode=Floor  overflowMode=off  firstCoeffDataTypeStr=Inherit: Same word length as input  firstCoeffMin=[]  firstCoeffMax=[]  firstCoeffLastDataTypeStr=Inherit: Same word length as input  outputDataTypeStr=Inherit: Same as accumulator  outputMin=[]  outputMax=[]  outputLastDataTypeStr=Inherit: Same as accumulator
  Freq1 : Constant  Value=2.4e6
  Mixer1 : Subsystem
  Real-Imag to Complex : RealImagToComplex
  Out1 : Outport
  wires:
  Constant/1 -> FIR Dec1/2
  Complex to Real-Imag/1 -> Mixer1/1(Input_I)
  Complex to Real-Imag1/1 -> Mixer1/3(DDS_I)
  Mixer1/2(Output_Q) -> Real-Imag to Complex/2
  Freq1/1 -> DDS_Gen1/1(In1)
  Complex to Real-Imag/2 -> Mixer1/2(Input_Q)
  Complex to Real-Imag1/2 -> Mixer1/4(DDS_Q)
  DDS_Gen1/1(Out1) -> Complex to Real-Imag1/1
  Real-Imag to Complex/1 -> FIR Dec1/1
  Mixer1/1(Output_I) -> Real-Imag to Complex/1
  FIR Dec1/1 -> Out1/1
  <IQ>/1 -> Complex to Real-Imag/1

== system Model/CORE_3_8/Path6 ==
  <IQ> : Inport
  Complex to Real-Imag : ComplexToRealImag
  Complex to Real-Imag1 : ComplexToRealImag
  Constant : Constant  Value=C12  SampleTime=dt0
  DDS_Gen1 : Subsystem
  FIR Dec1 : dspmlti4/FIR Decimation  FilterSource=Input port  h=designMultirateFIR(1,2)  D=2  filtStruct=Direct form  FilterObject=FDECIM  framing=Allow multirate processing  inputOffset=0  outputBufInitCond=0  roundingMode=Floor  overflowMode=off  firstCoeffDataTypeStr=Inherit: Same word length as input  firstCoeffMin=[]  firstCoeffMax=[]  firstCoeffLastDataTypeStr=Inherit: Same word length as input  outputDataTypeStr=Inherit: Same as accumulator  outputMin=[]  outputMax=[]  outputLastDataTypeStr=Inherit: Same as accumulator
  Freq1 : Constant  Value=2.4e6
  Mixer1 : Subsystem
  Real-Imag to Complex : RealImagToComplex
  Out1 : Outport
  wires:
  Constant/1 -> FIR Dec1/2
  Complex to Real-Imag/1 -> Mixer1/1(Input_I)
  Complex to Real-Imag1/1 -> Mixer1/3(DDS_I)
  Mixer1/2(Output_Q) -> Real-Imag to Complex/2
  Freq1/1 -> DDS_Gen1/1(In1)
  Complex to Real-Imag/2 -> Mixer1/2(Input_Q)
  Complex to Real-Imag1/2 -> Mixer1/4(DDS_Q)
  DDS_Gen1/1(Out1) -> Complex to Real-Imag1/1
  Real-Imag to Complex/1 -> FIR Dec1/1
  Mixer1/1(Output_I) -> Real-Imag to Complex/1
  FIR Dec1/1 -> Out1/1
  <IQ>/1 -> Complex to Real-Imag/1

== system Model/CORE_3_8/Path7 ==
  <IQ> : Inport
  Complex to Real-Imag : ComplexToRealImag
  Complex to Real-Imag1 : ComplexToRealImag
  Constant : Constant  Value=C12  SampleTime=dt0
  DDS_Gen1 : Subsystem
  FIR Dec1 : dspmlti4/FIR Decimation  FilterSource=Input port  h=designMultirateFIR(1,2)  D=2  filtStruct=Direct form  FilterObject=FDECIM  framing=Allow multirate processing  inputOffset=0  outputBufInitCond=0  roundingMode=Floor  overflowMode=off  firstCoeffDataTypeStr=Inherit: Same word length as input  firstCoeffMin=[]  firstCoeffMax=[]  firstCoeffLastDataTypeStr=Inherit: Same word length as input  outputDataTypeStr=Inherit: Same as accumulator  outputMin=[]  outputMax=[]  outputLastDataTypeStr=Inherit: Same as accumulator
  Freq1 : Constant  Value=2.4e6
  Mixer1 : Subsystem
  Real-Imag to Complex : RealImagToComplex
  Out1 : Outport
  wires:
  Constant/1 -> FIR Dec1/2
  Complex to Real-Imag/1 -> Mixer1/1(Input_I)
  Complex to Real-Imag1/1 -> Mixer1/3(DDS_I)
  Mixer1/2(Output_Q) -> Real-Imag to Complex/2
  Freq1/1 -> DDS_Gen1/1(In1)
  Complex to Real-Imag/2 -> Mixer1/2(Input_Q)
  Complex to Real-Imag1/2 -> Mixer1/4(DDS_Q)
  DDS_Gen1/1(Out1) -> Complex to Real-Imag1/1
  Real-Imag to Complex/1 -> FIR Dec1/1
  Mixer1/1(Output_I) -> Real-Imag to Complex/1
  FIR Dec1/1 -> Out1/1
  <IQ>/1 -> Complex to Real-Imag/1

== system Model/CORE_3_8/Path8 ==
  <IQ> : Inport
  Complex to Real-Imag : ComplexToRealImag
  Complex to Real-Imag1 : ComplexToRealImag
  Constant : Constant  Value=C12  SampleTime=dt0
  DDS_Gen1 : Subsystem
  FIR Dec1 : dspmlti4/FIR Decimation  FilterSource=Input port  h=designMultirateFIR(1,2)  D=2  filtStruct=Direct form  FilterObject=FDECIM  framing=Allow multirate processing  inputOffset=0  outputBufInitCond=0  roundingMode=Floor  overflowMode=off  firstCoeffDataTypeStr=Inherit: Same word length as input  firstCoeffMin=[]  firstCoeffMax=[]  firstCoeffLastDataTypeStr=Inherit: Same word length as input  outputDataTypeStr=Inherit: Same as accumulator  outputMin=[]  outputMax=[]  outputLastDataTypeStr=Inherit: Same as accumulator
  Freq1 : Constant  Value=2.4e6
  Mixer1 : Subsystem
  Real-Imag to Complex : RealImagToComplex
  Out1 : Outport
  wires:
  Constant/1 -> FIR Dec1/2
  Complex to Real-Imag/1 -> Mixer1/1(Input_I)
  Complex to Real-Imag1/1 -> Mixer1/3(DDS_I)
  Mixer1/2(Output_Q) -> Real-Imag to Complex/2
  Freq1/1 -> DDS_Gen1/1(In1)
  Complex to Real-Imag/2 -> Mixer1/2(Input_Q)
  Complex to Real-Imag1/2 -> Mixer1/4(DDS_Q)
  DDS_Gen1/1(Out1) -> Complex to Real-Imag1/1
  Real-Imag to Complex/1 -> FIR Dec1/1
  Mixer1/1(Output_I) -> Real-Imag to Complex/1
  FIR Dec1/1 -> Out1/1
  <IQ>/1 -> Complex to Real-Imag/1

== system Model/CORE_3_9/Path1 ==
  <IQ> : Inport
  Complex to Real-Imag : ComplexToRealImag
  Complex to Real-Imag1 : ComplexToRealImag
  Constant : Constant  Value=C12  SampleTime=dt0
  DDS_Gen1 : Subsystem
  FIR Dec1 : dspmlti4/FIR Decimation  FilterSource=Input port  h=designMultirateFIR(1,2)  D=2  filtStruct=Direct form  FilterObject=FDECIM  framing=Allow multirate processing  inputOffset=0  outputBufInitCond=0  roundingMode=Floor  overflowMode=off  firstCoeffDataTypeStr=Inherit: Same word length as input  firstCoeffMin=[]  firstCoeffMax=[]  firstCoeffLastDataTypeStr=Inherit: Same word length as input  outputDataTypeStr=Inherit: Same as accumulator  outputMin=[]  outputMax=[]  outputLastDataTypeStr=Inherit: Same as accumulator
  Freq1 : Constant  Value=2.4e6
  Mixer1 : Subsystem
  Real-Imag to Complex : RealImagToComplex
  Out1 : Outport
  wires:
  Constant/1 -> FIR Dec1/2
  Complex to Real-Imag/1 -> Mixer1/1(Input_I)
  Complex to Real-Imag1/1 -> Mixer1/3(DDS_I)
  Mixer1/2(Output_Q) -> Real-Imag to Complex/2
  Freq1/1 -> DDS_Gen1/1(In1)
  Complex to Real-Imag/2 -> Mixer1/2(Input_Q)
  Complex to Real-Imag1/2 -> Mixer1/4(DDS_Q)
  DDS_Gen1/1(Out1) -> Complex to Real-Imag1/1
  Real-Imag to Complex/1 -> FIR Dec1/1
  Mixer1/1(Output_I) -> Real-Imag to Complex/1
  FIR Dec1/1 -> Out1/1
  <IQ>/1 -> Complex to Real-Imag/1

== system Model/CORE_3_9/Path2 ==
  <IQ> : Inport
  Complex to Real-Imag : ComplexToRealImag
  Complex to Real-Imag1 : ComplexToRealImag
  Constant : Constant  Value=C12  SampleTime=dt0
  DDS_Gen1 : Subsystem
  FIR Dec1 : dspmlti4/FIR Decimation  FilterSource=Input port  h=designMultirateFIR(1,2)  D=2  filtStruct=Direct form  FilterObject=FDECIM  framing=Allow multirate processing  inputOffset=0  outputBufInitCond=0  roundingMode=Floor  overflowMode=off  firstCoeffDataTypeStr=Inherit: Same word length as input  firstCoeffMin=[]  firstCoeffMax=[]  firstCoeffLastDataTypeStr=Inherit: Same word length as input  outputDataTypeStr=Inherit: Same as accumulator  outputMin=[]  outputMax=[]  outputLastDataTypeStr=Inherit: Same as accumulator
  Freq1 : Constant  Value=2.4e6
  Mixer1 : Subsystem
  Real-Imag to Complex : RealImagToComplex
  Out1 : Outport
  wires:
  Constant/1 -> FIR Dec1/2
  Complex to Real-Imag/1 -> Mixer1/1(Input_I)
  Complex to Real-Imag1/1 -> Mixer1/3(DDS_I)
  Mixer1/2(Output_Q) -> Real-Imag to Complex/2
  Freq1/1 -> DDS_Gen1/1(In1)
  Complex to Real-Imag/2 -> Mixer1/2(Input_Q)
  Complex to Real-Imag1/2 -> Mixer1/4(DDS_Q)
  DDS_Gen1/1(Out1) -> Complex to Real-Imag1/1
  Real-Imag to Complex/1 -> FIR Dec1/1
  Mixer1/1(Output_I) -> Real-Imag to Complex/1
  FIR Dec1/1 -> Out1/1
  <IQ>/1 -> Complex to Real-Imag/1

== system Model/CORE_3_9/Path3 ==
  <IQ> : Inport
  Complex to Real-Imag : ComplexToRealImag
  Complex to Real-Imag1 : ComplexToRealImag
  Constant : Constant  Value=C12  SampleTime=dt0
  DDS_Gen1 : Subsystem
  FIR Dec1 : dspmlti4/FIR Decimation  FilterSource=Input port  h=designMultirateFIR(1,2)  D=2  filtStruct=Direct form  FilterObject=FDECIM  framing=Allow multirate processing  inputOffset=0  outputBufInitCond=0  roundingMode=Floor  overflowMode=off  firstCoeffDataTypeStr=Inherit: Same word length as input  firstCoeffMin=[]  firstCoeffMax=[]  firstCoeffLastDataTypeStr=Inherit: Same word length as input  outputDataTypeStr=Inherit: Same as accumulator  outputMin=[]  outputMax=[]  outputLastDataTypeStr=Inherit: Same as accumulator
  Freq1 : Constant  Value=2.4e6
  Mixer1 : Subsystem
  Real-Imag to Complex : RealImagToComplex
  Out1 : Outport
  wires:
  Constant/1 -> FIR Dec1/2
  Complex to Real-Imag/1 -> Mixer1/1(Input_I)
  Complex to Real-Imag1/1 -> Mixer1/3(DDS_I)
  Mixer1/2(Output_Q) -> Real-Imag to Complex/2
  Freq1/1 -> DDS_Gen1/1(In1)
  Complex to Real-Imag/2 -> Mixer1/2(Input_Q)
  Complex to Real-Imag1/2 -> Mixer1/4(DDS_Q)
  DDS_Gen1/1(Out1) -> Complex to Real-Imag1/1
  Real-Imag to Complex/1 -> FIR Dec1/1
  Mixer1/1(Output_I) -> Real-Imag to Complex/1
  FIR Dec1/1 -> Out1/1
  <IQ>/1 -> Complex to Real-Imag/1

== system Model/CORE_3_9/Path4 ==
  <IQ> : Inport
  Complex to Real-Imag : ComplexToRealImag
  Complex to Real-Imag1 : ComplexToRealImag
  Constant : Constant  Value=C12  SampleTime=dt0
  DDS_Gen1 : Subsystem
  FIR Dec1 : dspmlti4/FIR Decimation  FilterSource=Input port  h=designMultirateFIR(1,2)  D=2  filtStruct=Direct form  FilterObject=FDECIM  framing=Allow multirate processing  inputOffset=0  outputBufInitCond=0  roundingMode=Floor  overflowMode=off  firstCoeffDataTypeStr=Inherit: Same word length as input  firstCoeffMin=[]  firstCoeffMax=[]  firstCoeffLastDataTypeStr=Inherit: Same word length as input  outputDataTypeStr=Inherit: Same as accumulator  outputMin=[]  outputMax=[]  outputLastDataTypeStr=Inherit: Same as accumulator
  Freq1 : Constant  Value=2.4e6
  Mixer1 : Subsystem
  Real-Imag to Complex : RealImagToComplex
  Out1 : Outport
  wires:
  Constant/1 -> FIR Dec1/2
  Complex to Real-Imag/1 -> Mixer1/1(Input_I)
  Complex to Real-Imag1/1 -> Mixer1/3(DDS_I)
  Mixer1/2(Output_Q) -> Real-Imag to Complex/2
  Freq1/1 -> DDS_Gen1/1(In1)
  Complex to Real-Imag/2 -> Mixer1/2(Input_Q)
  Complex to Real-Imag1/2 -> Mixer1/4(DDS_Q)
  DDS_Gen1/1(Out1) -> Complex to Real-Imag1/1
  Real-Imag to Complex/1 -> FIR Dec1/1
  Mixer1/1(Output_I) -> Real-Imag to Complex/1
  FIR Dec1/1 -> Out1/1
  <IQ>/1 -> Complex to Real-Imag/1

== system Model/CORE_3_9/Path5 ==
  <IQ> : Inport
  Complex to Real-Imag : ComplexToRealImag
  Complex to Real-Imag1 : ComplexToRealImag
  Constant : Constant  Value=C12  SampleTime=dt0
  DDS_Gen1 : Subsystem
  FIR Dec1 : dspmlti4/FIR Decimation  FilterSource=Input port  h=designMultirateFIR(1,2)  D=2  filtStruct=Direct form  FilterObject=FDECIM  framing=Allow multirate processing  inputOffset=0  outputBufInitCond=0  roundingMode=Floor  overflowMode=off  firstCoeffDataTypeStr=Inherit: Same word length as input  firstCoeffMin=[]  firstCoeffMax=[]  firstCoeffLastDataTypeStr=Inherit: Same word length as input  outputDataTypeStr=Inherit: Same as accumulator  outputMin=[]  outputMax=[]  outputLastDataTypeStr=Inherit: Same as accumulator
  Freq1 : Constant  Value=2.4e6
  Mixer1 : Subsystem
  Real-Imag to Complex : RealImagToComplex
  Out1 : Outport
  wires:
  Constant/1 -> FIR Dec1/2
  Complex to Real-Imag/1 -> Mixer1/1(Input_I)
  Complex to Real-Imag1/1 -> Mixer1/3(DDS_I)
  Mixer1/2(Output_Q) -> Real-Imag to Complex/2
  Freq1/1 -> DDS_Gen1/1(In1)
  Complex to Real-Imag/2 -> Mixer1/2(Input_Q)
  Complex to Real-Imag1/2 -> Mixer1/4(DDS_Q)
  DDS_Gen1/1(Out1) -> Complex to Real-Imag1/1
  Real-Imag to Complex/1 -> FIR Dec1/1
  Mixer1/1(Output_I) -> Real-Imag to Complex/1
  FIR Dec1/1 -> Out1/1
  <IQ>/1 -> Complex to Real-Imag/1

== system Model/CORE_3_9/Path6 ==
  <IQ> : Inport
  Complex to Real-Imag : ComplexToRealImag
  Complex to Real-Imag1 : ComplexToRealImag
  Constant : Constant  Value=C12  SampleTime=dt0
  DDS_Gen1 : Subsystem
  FIR Dec1 : dspmlti4/FIR Decimation  FilterSource=Input port  h=designMultirateFIR(1,2)  D=2  filtStruct=Direct form  FilterObject=FDECIM  framing=Allow multirate processing  inputOffset=0  outputBufInitCond=0  roundingMode=Floor  overflowMode=off  firstCoeffDataTypeStr=Inherit: Same word length as input  firstCoeffMin=[]  firstCoeffMax=[]  firstCoeffLastDataTypeStr=Inherit: Same word length as input  outputDataTypeStr=Inherit: Same as accumulator  outputMin=[]  outputMax=[]  outputLastDataTypeStr=Inherit: Same as accumulator
  Freq1 : Constant  Value=2.4e6
  Mixer1 : Subsystem
  Real-Imag to Complex : RealImagToComplex
  Out1 : Outport
  wires:
  Constant/1 -> FIR Dec1/2
  Complex to Real-Imag/1 -> Mixer1/1(Input_I)
  Complex to Real-Imag1/1 -> Mixer1/3(DDS_I)
  Mixer1/2(Output_Q) -> Real-Imag to Complex/2
  Freq1/1 -> DDS_Gen1/1(In1)
  Complex to Real-Imag/2 -> Mixer1/2(Input_Q)
  Complex to Real-Imag1/2 -> Mixer1/4(DDS_Q)
  DDS_Gen1/1(Out1) -> Complex to Real-Imag1/1
  Real-Imag to Complex/1 -> FIR Dec1/1
  Mixer1/1(Output_I) -> Real-Imag to Complex/1
  FIR Dec1/1 -> Out1/1
  <IQ>/1 -> Complex to Real-Imag/1

== system Model/CORE_3_9/Path7 ==
  <IQ> : Inport
  Complex to Real-Imag : ComplexToRealImag
  Complex to Real-Imag1 : ComplexToRealImag
  Constant : Constant  Value=C12  SampleTime=dt0
  DDS_Gen1 : Subsystem
  FIR Dec1 : dspmlti4/FIR Decimation  FilterSource=Input port  h=designMultirateFIR(1,2)  D=2  filtStruct=Direct form  FilterObject=FDECIM  framing=Allow multirate processing  inputOffset=0  outputBufInitCond=0  roundingMode=Floor  overflowMode=off  firstCoeffDataTypeStr=Inherit: Same word length as input  firstCoeffMin=[]  firstCoeffMax=[]  firstCoeffLastDataTypeStr=Inherit: Same word length as input  outputDataTypeStr=Inherit: Same as accumulator  outputMin=[]  outputMax=[]  outputLastDataTypeStr=Inherit: Same as accumulator
  Freq1 : Constant  Value=2.4e6
  Mixer1 : Subsystem
  Real-Imag to Complex : RealImagToComplex
  Out1 : Outport
  wires:
  Constant/1 -> FIR Dec1/2
  Complex to Real-Imag/1 -> Mixer1/1(Input_I)
  Complex to Real-Imag1/1 -> Mixer1/3(DDS_I)
  Mixer1/2(Output_Q) -> Real-Imag to Complex/2
  Freq1/1 -> DDS_Gen1/1(In1)
  Complex to Real-Imag/2 -> Mixer1/2(Input_Q)
  Complex to Real-Imag1/2 -> Mixer1/4(DDS_Q)
  DDS_Gen1/1(Out1) -> Complex to Real-Imag1/1
  Real-Imag to Complex/1 -> FIR Dec1/1
  Mixer1/1(Output_I) -> Real-Imag to Complex/1
  FIR Dec1/1 -> Out1/1
  <IQ>/1 -> Complex to Real-Imag/1

== system Model/CORE_3_9/Path8 ==
  <IQ> : Inport
  Complex to Real-Imag : ComplexToRealImag
  Complex to Real-Imag1 : ComplexToRealImag
  Constant : Constant  Value=C12  SampleTime=dt0
  DDS_Gen1 : Subsystem
  FIR Dec1 : dspmlti4/FIR Decimation  FilterSource=Input port  h=designMultirateFIR(1,2)  D=2  filtStruct=Direct form  FilterObject=FDECIM  framing=Allow multirate processing  inputOffset=0  outputBufInitCond=0  roundingMode=Floor  overflowMode=off  firstCoeffDataTypeStr=Inherit: Same word length as input  firstCoeffMin=[]  firstCoeffMax=[]  firstCoeffLastDataTypeStr=Inherit: Same word length as input  outputDataTypeStr=Inherit: Same as accumulator  outputMin=[]  outputMax=[]  outputLastDataTypeStr=Inherit: Same as accumulator
  Freq1 : Constant  Value=2.4e6
  Mixer1 : Subsystem
  Real-Imag to Complex : RealImagToComplex
  Out1 : Outport
  wires:
  Constant/1 -> FIR Dec1/2
  Complex to Real-Imag/1 -> Mixer1/1(Input_I)
  Complex to Real-Imag1/1 -> Mixer1/3(DDS_I)
  Mixer1/2(Output_Q) -> Real-Imag to Complex/2
  Freq1/1 -> DDS_Gen1/1(In1)
  Complex to Real-Imag/2 -> Mixer1/2(Input_Q)
  Complex to Real-Imag1/2 -> Mixer1/4(DDS_Q)
  DDS_Gen1/1(Out1) -> Complex to Real-Imag1/1
  Real-Imag to Complex/1 -> FIR Dec1/1
  Mixer1/1(Output_I) -> Real-Imag to Complex/1
  FIR Dec1/1 -> Out1/1
  <IQ>/1 -> Complex to Real-Imag/1

== system Model/CORE_3_1/Path1/DDS_Gen1 ==
  In1 : Inport
  Exp : Math  SaturateOnIntegerOverflow=on
  Gain : Gain  Gain=-1i*2*pi
  Product : Product
  Signal From Workspace1 : dspsrcs4/Signal From Workspace  X=t0  Ts=dt0  nsamps=1  OutputAfterFinalValue=Cyclic repetition  ignoreOrWarnInputAndFrameLengths=off  OutputFrames=off
  Out1 : Outport
  wires:
  Signal From Workspace1/1 -> Gain/1
  Exp/1 -> Out1/1
  Gain/1 -> Product/2
  Product/1 -> Exp/1
  In1/1 -> Product/1
